simulink model "test_ctrl"  (R2023a)
settings: Solver=FixedStepAuto  StartTime=0.0  StopTime=Inf  RelTol=1e-3  EnableMultiTasking=on
undefined symbols (not defined in the file): Green, led0
libraries: embedlinuxNetworklib x2, simulink x1, raspberrypiBasiclib x1, embmathops x1
settings Model: SimulationMode=external  ExtModeTrigDuration=2  Creator=gabor  LastModifiedBy=umphaipunatipunumphai
settings SolverCC: AlgebraicLoopSolver=TrustRegion  PositivePriorityOrder=on
settings DataIOCC: InspectSignalLogs=on
settings OptimizationCC: EnhancedBackFolding=on  PassReuseOutputArgsAs=Individual arguments  ZeroExternalMemoryAtStartup=off  ZeroInternalMemoryAtStartup=off  MaxStackSize=64  OptimizeBlockOrder=speed  DifferentSizesBufferReuse=on  OptimizationCustomize=off  EfficientTunableParamExpr=on
settings DebuggingCC: ParameterTunabilityLossMsg=error  UnconnectedInputMsg=warning  UnconnectedOutputMsg=warning  UnconnectedLineMsg=warning
settings HardwareCC: ProdBitPerPointer=32  ProdBitPerSizeT=32  ProdBitPerPtrDiffT=32  ProdLargestAtomicInteger=Long  ProdLargestAtomicFloat=Double  ProdWordSize=32  ProdLongLongMode=on  ProdHWDeviceType=ARM Compatible->ARM Cortex
settings ModelReferenceCC: EnableRefExpFcnMdlSchedulingChecks=on
settings RTWCC: Description=Embedded Coder  SystemTargetFile=ert.tlc  HardwareBoard=Raspberry Pi  TLCOptions="-aInlineSetEventsForThisBaseRateFcn=TLC_FALSE -aSuppressMultiTaskScheduler=TLC_FALSE  -aRateBasedStepFcn=0"  TemplateMakefile=ert_default_tmf  Toolchain=GNU GCC Embedded Linux  BuildConfiguration=Faster Runs  DLArmComputeVersion=19.05
settings CodeAppCC: ForceParamTrailComments=on  IgnoreCustomStorageClasses=off  OperatorAnnotations=on  SimulinkDataObjDesc=on  SFDataObjDesc=on  InsertBlockDesc=on
settings ERTTargetCC: SupportVariableSizeSignals=on  ExtModeTransport=2  ExtModeStaticAlloc=on  ExtModeMexFile=ext_xcp  ExtModeIntrfLevel=Level2 - Open

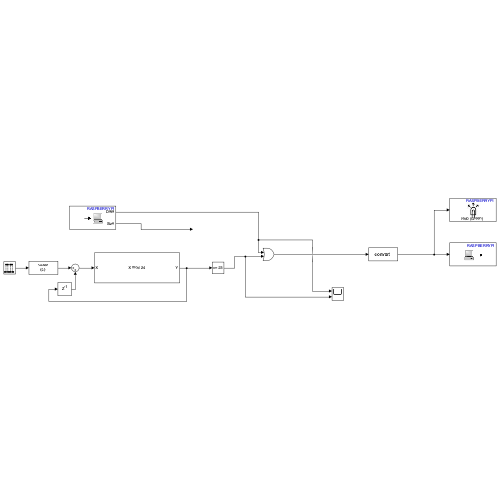
[thumbnail: Simulink's stored preview of the top-level diagram]
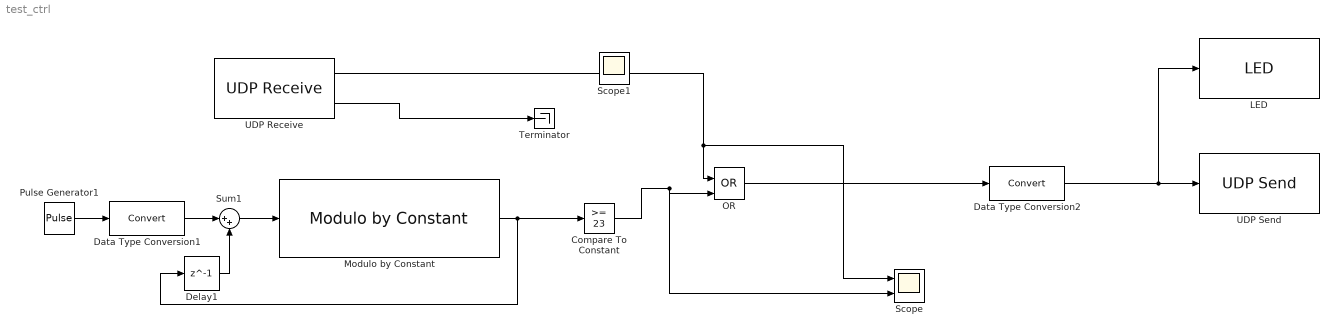
== system test_ctrl ==
  Compare To Constant : simulink/Logic and Bit Operations/Compare To Constant  relop=>=  const=23  OutDataTypeStr=boolean
  Data Type Conversion1 : DataTypeConversion  OutMin=0  OutMax=1  ConvertRealWorld=Stored Integer (SI)  RndMeth=Nearest  SaturateOnIntegerOverflow=off
  Data Type Conversion2 : DataTypeConversion  SaturateOnIntegerOverflow=off  RndMeth=Floor
  Delay1 : Delay  DelayLength=1  InitialCondition=0  SampleTime=1
  LED : raspberrypiBasiclib/LED  BoardProperty=Pi 3 Model B+  LED_=led0 (Green)
  Modulo by Constant : embmathops/Modulo by Constant  Denominator=24  SimulateUsing=Code generation
      settings: LibrarySourceBlock=embeddedMathLib/Modulo by Constant
  OR : Logic  Operator=OR  IconShape=distinctive  AllPortsSameDT=off  OutDataTypeStr=boolean
  Pulse Generator1 : DiscretePulseGenerator  Period=10  PulseWidth=5
  Scope : Scope  NumInputPorts=2
  Sum1 : Sum  Inputs=|++
  Terminator : Terminator
  UDP Receive : embedlinuxNetworklib/UDP Receive  localURL='0.0.0.0'  localPort=25000  remoteURL='0.0.0.0'  remotePort=-1  recvBufferSize=8192  signalDatatype=double  dims=1  isVarSize=off  showBlockingTime=off  blockingTime=0  sampletime=1.0  blockPlatform=Raspberry Pi
  UDP Send : embedlinuxNetworklib/UDP Send  remoteURL='192.168.137.1'  remotePort=26000  localURL='0.0.0.0'  localPortSource=Automatically determine  localPort=-1  sampletime=-1  blockPlatform=Raspberry Pi  separateLengthPort=0
  Scope1 : Scope
  wires:
  UDP Receive/2 -> Terminator/1
  Compare To Constant/1 -> Scope/2, OR/2
  Data Type Conversion2/1 -> LED/1, UDP Send/1
  Data Type Conversion1/1 -> Sum1/1
  Sum1/1 -> Modulo by Constant/1
  Delay1/1 -> Sum1/2
  Pulse Generator1/1 -> Data Type Conversion1/1
  OR/1 -> Data Type Conversion2/1
  Modulo by Constant/1 -> Compare To Constant/1, Delay1/1
  UDP Receive/1 -> OR/1, Scope/1
